simulink model "SMD"  (R2015b)
settings: Solver=VariableStepAuto  StartTime=0.0  StopTime=10.0  RelTol=1e-3
undefined symbols (not defined in the file): a, alpha, alpha_not, alpha_one, b, beta, c, Csfl, Csfr, Csfrl, Csrl, Csrr, d, gama, Ixx, Iyy, Ksfl, Ksfr, Ksrl, Ksrr, Kufl, Kufr, Kurl, Kurr, lamda_not, lamda_one, M, m, Ps, S, tao, Ufl, Ufr, Url, Urr
settings Model: Creator=Guest  LastModifiedBy=Guest

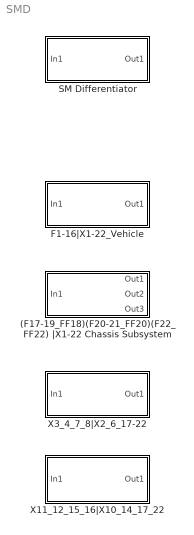
== system SMD ==
  "(F17-19_FF18)(F20-21_FF20)(F22_FF22) |X1-22 Chassis Subsystem " : Subsystem  TreatAsAtomicUnit=on
  "F1-16|X1-22_Vehicle " : Subsystem  TreatAsAtomicUnit=on
  "SM Differentiator " : Subsystem  TreatAsAtomicUnit=on
  X11_12_15_16|X10_14_17_22 : Subsystem  TreatAsAtomicUnit=on
  X3_4_7_8|X2_6_17-22 : Subsystem  TreatAsAtomicUnit=on

== system SMD/(F17-19_FF18)(F20-21_FF20)(F22_FF22) |X1-22 Chassis Subsystem  ==
  In1 : Inport
  F17_18_19_FF18|X1_22 : Subsystem  TreatAsAtomicUnit=on
  "F20_21_FF20|X1_22 " : Subsystem  TreatAsAtomicUnit=on
  F22_FF22|X1_22 : Subsystem  TreatAsAtomicUnit=on
  Out1 : Outport
  Out2 : Outport  Port=2
  Out3 : Outport  Port=3
  wires:
  In1/1 -> F17_18_19_FF18|X1_22/1(In1), "F20_21_FF20|X1_22 "/1(In1), F22_FF22|X1_22/1(In1)
  F22_FF22|X1_22/1(Out1) -> Out3/1
  "F20_21_FF20|X1_22 "/1(Out1) -> Out2/1
  F17_18_19_FF18|X1_22/1(Out1) -> Out1/1

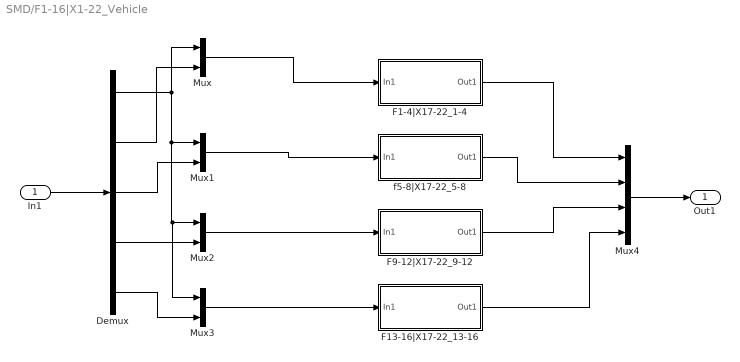
== system SMD/F1-16|X1-22_Vehicle  ==
  In1 : Inport
  Demux : Demux  Outputs=5
  F1-4|X17-22_1-4 : Subsystem  TreatAsAtomicUnit=on
  F13-16|X17-22_13-16 : Subsystem  TreatAsAtomicUnit=on
  F9-12|X17-22_9-12 : Subsystem  TreatAsAtomicUnit=on
  Mux{,1..3} (4 alike) : Mux  Inputs=2
  Mux4 : Mux
  f5-8|X17-22_5-8 : Subsystem  TreatAsAtomicUnit=on
  Out1 : Outport
  wires:
  Demux/1 -> Mux3/1, Mux2/1, Mux1/1, Mux/1
  Demux/2 -> Mux/2
  Mux/1 -> F1-4|X17-22_1-4/1(In1)
  Demux/3 -> Mux1/2
  Mux1/1 -> f5-8|X17-22_5-8/1(In1)
  Demux/4 -> Mux2/2
  Mux2/1 -> F9-12|X17-22_9-12/1(In1)
  Mux3/1 -> F13-16|X17-22_13-16/1(In1)
  Demux/5 -> Mux3/2
  In1/1 -> Demux/1
  F1-4|X17-22_1-4/1(Out1) -> Mux4/1
  f5-8|X17-22_5-8/1(Out1) -> Mux4/2
  F9-12|X17-22_9-12/1(Out1) -> Mux4/3
  F13-16|X17-22_13-16/1(Out1) -> Mux4/4
  Mux4/1 -> Out1/1

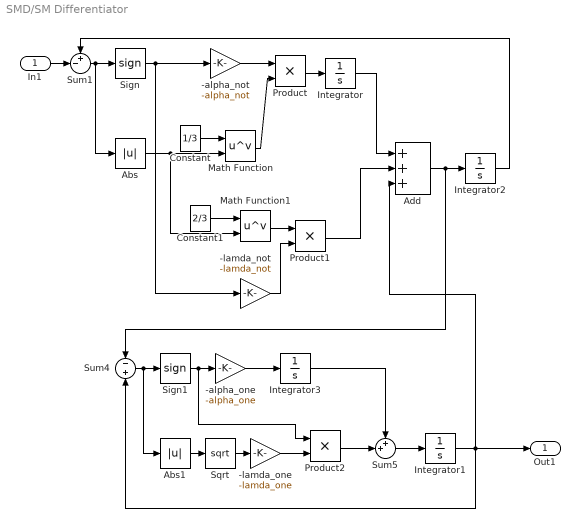
== system SMD/SM Differentiator  ==
  In1 : Inport
  "-alpha_not " : Gain  Gain=-alpha_not
  "-alpha_one " : Gain  Gain=-alpha_one
  "-lamda_not " : Gain  Gain=-lamda_not
  "-lamda_one " : Gain  Gain=-lamda_one
  Abs : Abs
  Abs1 : Abs
  Add : Sum  Inputs=+++
  Constant : Constant  Value=1/3
  Constant1 : Constant  Value=2/3
  Integrator{,1..3} (4 alike) : Integrator
  Math Function : Math  Operator=pow  SaturateOnIntegerOverflow=on
  Math Function1 : Math  Operator=pow  SaturateOnIntegerOverflow=on
  Product : Product
  Product1 : Product
  Product2 : Product
  Sign : Signum
  Sign1 : Signum
  Sqrt : Sqrt  SaturateOnIntegerOverflow=on
  Sum1 : Sum  Inputs=+-|
  Sum4 : Sum  Inputs=-|+
  Sum5 : Sum  Inputs=++|
  Out1 : Outport
  wires:
  Sum1/1 -> Abs/1, Sign/1
  Abs/1 -> Math Function1/2, Math Function/2
  "-alpha_not "/1 -> Product/1
  Constant/1 -> Math Function/1
  Math Function/1 -> Product/2
  Sign/1 -> "-lamda_not "/1, "-alpha_not "/1
  Product/1 -> Integrator/1
  Constant1/1 -> Math Function1/1
  Math Function1/1 -> Product1/1
  "-lamda_not "/1 -> Product1/2
  Integrator/1 -> Add/1
  Product1/1 -> Add/2
  Add/1 -> Sum4/1, Integrator2/1
  Integrator2/1 -> Sum1/1
  Sum4/1 -> Abs1/1, Sign1/1
  Sign1/1 -> Product2/1, "-alpha_one "/1
  "-alpha_one "/1 -> Integrator3/1
  Abs1/1 -> Sqrt/1
  Sqrt/1 -> "-lamda_one "/1
  "-lamda_one "/1 -> Product2/2
  Product2/1 -> Sum5/2
  Integrator3/1 -> Sum5/1
  Sum5/1 -> Integrator1/1
  Integrator1/1 -> Out1/1, Sum4/2, Add/3
  In1/1 -> Sum1/2

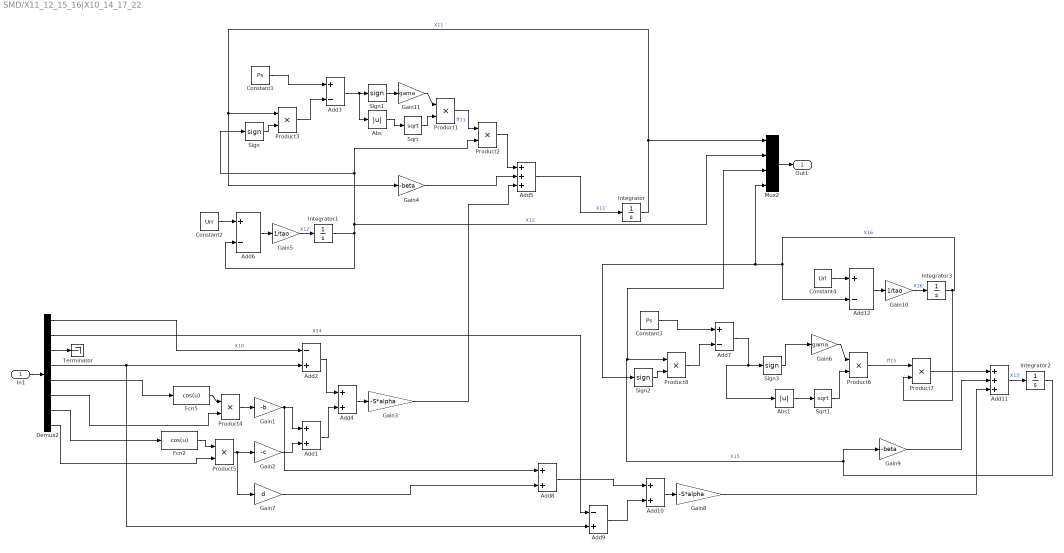
== system SMD/X11_12_15_16|X10_14_17_22 ==
  In1 : Inport
  Abs : Abs
  Abs1 : Abs
  Add{1,4,8,10} (4 alike) : Sum
  Add11 : Sum  Inputs=+++
  Add{3,6..7,12} (4 alike) : Sum  Inputs=+-
  Add2 : Sum  Inputs=-+
  Add5 : Sum  Inputs=+++
  Add9 : Sum  Inputs=-+
  Constant1 : Constant  Value=Ps
  Constant2 : Constant  Value=Urr
  Constant3 : Constant  Value=Ps
  Constant4 : Constant  Value=Url
  Demux2 : Demux  Outputs=8
  Fcn2 : Fcn  Expr=cos(u)
  Fcn5 : Fcn  Expr=cos(u)
  Gain1 : Gain  Gain=-b
  Gain10 : Gain  Gain=1/tao
  Gain11 : Gain  Gain=gama
  Gain2 : Gain  Gain=-c
  Gain3 : Gain  Gain=-S*alpha
  Gain4 : Gain  Gain=-beta
  Gain5 : Gain  Gain=1/tao
  Gain6 : Gain  Gain=gama
  Gain7 : Gain  Gain=d
  Gain8 : Gain  Gain=-S*alpha
  Gain9 : Gain  Gain=-beta
  Integrator{,1..3} (4 alike) : Integrator
  Mux2 : Mux
  Product{1..8} (8 alike) : Product
  Sign{,1..3} (4 alike) : Signum
  Sqrt : Sqrt  SaturateOnIntegerOverflow=on
  Sqrt1 : Sqrt  SaturateOnIntegerOverflow=on
  Terminator : Terminator
  Out1 : Outport
  wires:
  Constant1/1 -> Add3/1
  Product3/1 -> Add3/2
  Add3/1 -> Abs/1, Sign1/1
  Sign1/1 -> Gain11/1
  Abs/1 -> Sqrt/1
  Gain11/1 -> Product1/1
  Sqrt/1 -> Product1/2
  Sign/1 -> Product3/2
  Product1/1 -> Product2/1  "ff11"
  Demux2/5 -> Fcn5/1
  Fcn5/1 -> Product4/1
  Demux2/6 -> Product4/2
  Product4/1 -> Gain1/1
  Demux2/7 -> Fcn2/1
  Fcn2/1 -> Product5/1
  Demux2/8 -> Product5/2
  Product5/1 -> Gain7/1, Gain2/1
  Gain2/1 -> Add1/2
  Gain1/1 -> Add8/1, Add1/1
  Demux2/4 -> Add9/2, Add2/2
  Add2/1 -> Add4/1
  Add1/1 -> Add4/2
  Add4/1 -> Gain3/1
  Product2/1 -> Add5/1
  Gain4/1 -> Add5/2
  Gain3/1 -> Add5/3
  Add5/1 -> Integrator/1  "X11'"
  Integrator/1 -> Gain4/1, Product3/1, Mux2/1  "X11"
  Constant2/1 -> Add6/1
  Add6/1 -> Gain5/1
  Gain5/1 -> Integrator1/1  "X12'"
  Integrator1/1 -> Mux2/2, Sign/1, Product2/2, Add6/2  "X12"
  Constant3/1 -> Add7/1
  Product8/1 -> Add7/2
  Add7/1 -> Abs1/1, Sign3/1
  Sign3/1 -> Gain6/1
  Gain6/1 -> Product6/1
  Sqrt1/1 -> Product6/2
  Sign2/1 -> Product8/2
  Product6/1 -> Product7/1  "ff15"
  Abs1/1 -> Sqrt1/1
  Gain7/1 -> Add8/2
  Demux2/2 -> Add9/1  "X14"
  Add9/1 -> Add10/2
  Add8/1 -> Add10/1
  Add10/1 -> Gain8/1
  Product7/1 -> Add11/1
  Gain9/1 -> Add11/2
  Gain8/1 -> Add11/3
  Add11/1 -> Integrator2/1  "X15'"
  Integrator2/1 -> Mux2/3, Product8/1, Gain9/1  "X15"
  Constant4/1 -> Add12/1
  Add12/1 -> Gain10/1
  Gain10/1 -> Integrator3/1  "X16'"
  Integrator3/1 -> Product7/2, Mux2/4, Sign2/1, Add12/2  "X16"
  Demux2/1 -> Add2/1  "X10"
  Mux2/1 -> Out1/1
  In1/1 -> Demux2/1
  Demux2/3 -> Terminator/1

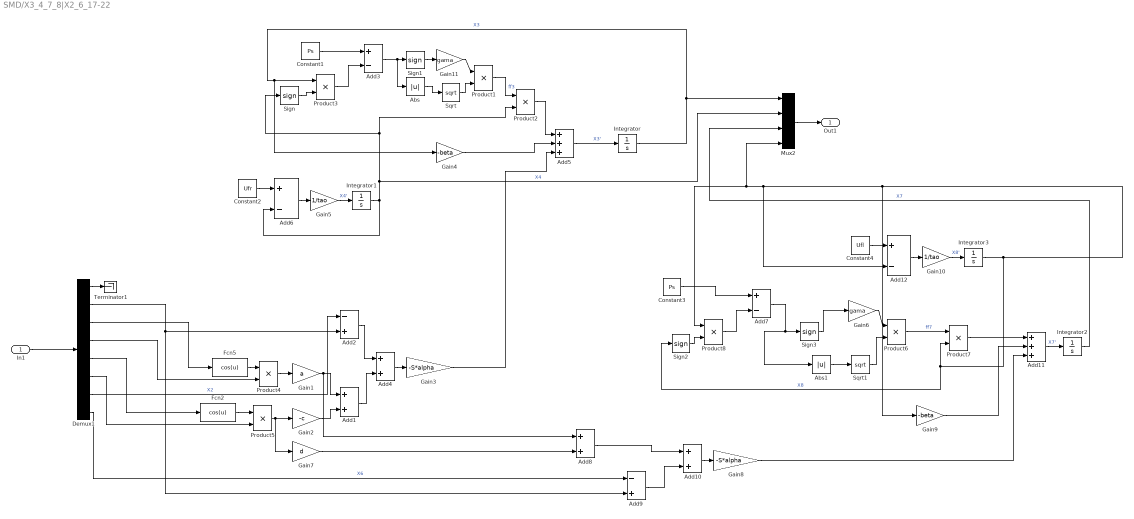
== system SMD/X3_4_7_8|X2_6_17-22 ==
  In1 : Inport
  Abs : Abs
  Abs1 : Abs
  Add{1,4,8,10} (4 alike) : Sum
  Add11 : Sum  Inputs=+++
  Add{3,6..7,12} (4 alike) : Sum  Inputs=+-
  Add2 : Sum  Inputs=-+
  Add5 : Sum  Inputs=+++
  Add9 : Sum  Inputs=-+
  Constant1 : Constant  Value=Ps
  Constant2 : Constant  Value=Ufr
  Constant3 : Constant  Value=Ps
  Constant4 : Constant  Value=Ufl
  Demux1 : Demux  Outputs=8
  Fcn2 : Fcn  Expr=cos(u)
  Fcn5 : Fcn  Expr=cos(u)
  Gain1 : Gain  Gain=a
  Gain10 : Gain  Gain=1/tao
  Gain11 : Gain  Gain=gama
  Gain2 : Gain  Gain=-c
  Gain3 : Gain  Gain=-S*alpha
  Gain4 : Gain  Gain=-beta
  Gain5 : Gain  Gain=1/tao
  Gain6 : Gain  Gain=gama
  Gain7 : Gain  Gain=d
  Gain8 : Gain  Gain=-S*alpha
  Gain9 : Gain  Gain=-beta
  Integrator{,1..3} (4 alike) : Integrator
  Mux2 : Mux
  Product{1..8} (8 alike) : Product
  Sign{,1..3} (4 alike) : Signum
  Sqrt : Sqrt  SaturateOnIntegerOverflow=on
  Sqrt1 : Sqrt  SaturateOnIntegerOverflow=on
  Terminator1 : Terminator
  Out1 : Outport
  wires:
  Constant1/1 -> Add3/1
  Product3/1 -> Add3/2
  Add3/1 -> Abs/1, Sign1/1
  Sign1/1 -> Gain11/1
  Abs/1 -> Sqrt/1
  Gain11/1 -> Product1/1
  Sqrt/1 -> Product1/2
  Sign/1 -> Product3/2
  Product1/1 -> Product2/1  "ff3"
  Demux1/3 -> Fcn5/1
  Fcn5/1 -> Product4/1
  Demux1/4 -> Product4/2
  Product4/1 -> Gain1/1
  Fcn2/1 -> Product5/1
  Product5/1 -> Gain7/1, Gain2/1
  Gain2/1 -> Add1/2
  Gain1/1 -> Add8/1, Add1/1
  Demux1/2 -> Add9/2, Add2/2
  Demux1/7 -> Add2/1  "X2"
  Add2/1 -> Add4/1
  Add1/1 -> Add4/2
  Add4/1 -> Gain3/1
  Product2/1 -> Add5/1
  Gain4/1 -> Add5/2
  Gain3/1 -> Add5/3
  Add5/1 -> Integrator/1  "X3'"
  Constant2/1 -> Add6/1
  Add6/1 -> Gain5/1
  Gain5/1 -> Integrator1/1  "X4'"
  Constant3/1 -> Add7/1
  Product8/1 -> Add7/2
  Add7/1 -> Abs1/1, Sign3/1
  Sign3/1 -> Gain6/1
  Gain6/1 -> Product6/1
  Sqrt1/1 -> Product6/2
  Sign2/1 -> Product8/2
  Product6/1 -> Product7/1  "ff7"
  Abs1/1 -> Sqrt1/1
  Gain7/1 -> Add8/2
  Add9/1 -> Add10/2
  Add8/1 -> Add10/1
  Add10/1 -> Gain8/1
  Product7/1 -> Add11/1
  Gain9/1 -> Add11/2
  Gain8/1 -> Add11/3
  Add11/1 -> Integrator2/1  "X7'"
  Integrator3/1 -> Product7/2, Sign2/1, Gain9/1, Add12/2, Product8/1, Mux2/4  "X8"
  Constant4/1 -> Add12/1
  Add12/1 -> Gain10/1
  Gain10/1 -> Integrator3/1  "X8'"
  Integrator2/1 -> Mux2/3  "X7"
  Integrator/1 -> Mux2/1, Gain4/1, Product3/1  "X3"
  Integrator1/1 -> Mux2/2, Sign/1, Product2/2, Add6/2  "X4"
  Demux1/8 -> Add9/1  "X6"
  In1/1 -> Demux1/1
  Mux2/1 -> Out1/1
  Demux1/1 -> Terminator1/1
  Demux1/5 -> Fcn2/1
  Demux1/6 -> Product5/2

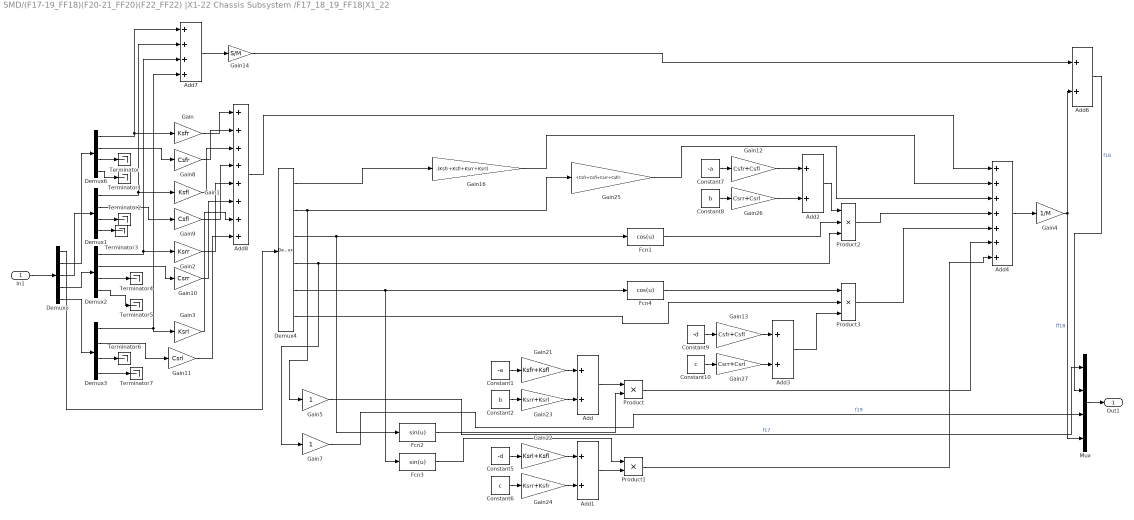
== system SMD/(F17-19_FF18)(F20-21_FF20)(F22_FF22) |X1-22 Chassis Subsystem /F17_18_19_FF18|X1_22 ==
  In1 : Inport
  Add{,1..3,6} (5 alike) : Sum
  Add4 : Sum  Inputs=+++++++
  Add7 : Sum  Inputs=++++
  Add8 : Sum  Inputs=++++++++
  Constant1 : Constant  Value=-a
  Constant10 : Constant  Value=c
  Constant2 : Constant  Value=b
  Constant5 : Constant  Value=-d
  Constant6 : Constant  Value=c
  Constant7 : Constant  Value=-a
  Constant8 : Constant  Value=b
  Constant9 : Constant  Value=-d
  Demux{1..3,6} (4 alike) : Demux
  Demux4 : Demux  Outputs=6
  Demux5 : Demux  Outputs=5
  Fcn1 : Fcn  Expr=cos(u)
  Fcn2 : Fcn  Expr=sin(u)
  Fcn3 : Fcn  Expr=sin(u)
  Fcn4 : Fcn  Expr=cos(u)
  Gain : Gain  Gain=Ksfr
  Gain1 : Gain  Gain=Ksfl
  Gain10 : Gain  Gain=Csrr
  Gain11 : Gain  Gain=Csrl
  Gain12 : Gain  Gain=Csfr+Csfl
  Gain13 : Gain  Gain=Csfr+Csfl
  Gain14 : Gain  Gain=S/M
  Gain16 : Gain  Gain=-(Ksfr+Ksfl+Ksrr+Ksrl)
  Gain2 : Gain  Gain=Ksrr
  Gain21 : Gain  Gain=Ksfr+Ksfl
  Gain22 : Gain  Gain=Ksrl+Ksfl
  Gain23 : Gain  Gain=Ksrr+Ksrl
  Gain24 : Gain  Gain=Ksrr+Ksfr
  Gain25 : Gain  Gain=-(Csfr+Csfl+Csrr+Csfr)
  Gain26 : Gain  Gain=Csrr+Csrl
  Gain27 : Gain  Gain=Csrr+Csrl
  Gain3 : Gain  Gain=Ksrl
  Gain4 : Gain  Gain=1/M
  Gain5 : Gain
  Gain7 : Gain
  Gain8 : Gain  Gain=Csfr
  Gain9 : Gain  Gain=Csfl
  Mux : Mux
  Product : Product
  Product1 : Product
  Product2 : Product  Inputs=3
  Product3 : Product  Inputs=3
  Terminator{,1..7} (8 alike) : Terminator
  Out1 : Outport
  wires:
  Demux6/1 -> Add7/1, Gain/1
  Demux1/1 -> Gain1/1, Add7/2
  Demux2/1 -> Gain2/1, Add7/3
  Demux3/1 -> Gain3/1, Add7/4
  Demux4/1 -> Gain16/1
  Demux4/3 -> Fcn2/1, Fcn1/1
  Gain21/1 -> Add/1
  Constant1/1 -> Gain21/1
  Gain23/1 -> Add/2
  Constant2/1 -> Gain23/1
  Add/1 -> Product/1
  Fcn2/1 -> Product/2
  Demux4/5 -> Fcn3/1, Fcn4/1
  Gain22/1 -> Add1/1
  Gain24/1 -> Add1/2
  Constant5/1 -> Gain22/1
  Constant6/1 -> Gain24/1
  Add1/1 -> Product1/2
  Fcn3/1 -> Product1/1
  Demux4/2 -> Gain5/1, Gain25/1
  Demux4/4 -> Gain7/1, Product2/3
  Fcn1/1 -> Product2/2
  Gain12/1 -> Add2/1
  Constant7/1 -> Gain12/1
  Gain26/1 -> Add2/2
  Constant8/1 -> Gain26/1
  Add2/1 -> Product2/1
  Gain13/1 -> Add3/1
  Constant9/1 -> Gain13/1
  Gain27/1 -> Add3/2
  Constant10/1 -> Gain27/1
  Fcn4/1 -> Product3/1
  Demux4/6 -> Product3/2
  Add3/1 -> Product3/3
  Product/1 -> Add4/6
  Product1/1 -> Add4/7
  Add4/1 -> Gain4/1
  Gain14/1 -> Add6/1
  Gain4/1 -> Add6/2, Mux/4  "ff18"
  Add6/1 -> Mux/2  "f18"
  Gain5/1 -> Mux/1  "f17"
  Gain7/1 -> Mux/3  "f19"
  Demux6/2 -> Gain8/1
  Demux1/2 -> Gain9/1
  Demux2/2 -> Gain10/1
  Demux3/2 -> Gain11/1
  Add7/1 -> Gain14/1
  Gain/1 -> Add8/1
  Gain8/1 -> Add8/2
  Gain1/1 -> Add8/3
  Gain9/1 -> Add8/4
  Gain2/1 -> Add8/5
  Gain10/1 -> Add8/6
  Gain3/1 -> Add8/7
  Gain11/1 -> Add8/8
  Product3/1 -> Add4/5
  Product2/1 -> Add4/4
  Gain25/1 -> Add4/3
  Gain16/1 -> Add4/2
  Add8/1 -> Add4/1
  Demux6/3 -> Terminator/1
  Demux6/4 -> Terminator1/1
  Demux1/3 -> Terminator2/1
  Demux1/4 -> Terminator3/1
  Demux2/3 -> Terminator4/1
  Demux2/4 -> Terminator5/1
  Demux3/3 -> Terminator6/1
  Demux3/4 -> Terminator7/1
  Demux5/2 -> Demux6/1
  Demux5/3 -> Demux1/1
  Demux5/4 -> Demux2/1
  Demux5/5 -> Demux3/1
  In1/1 -> Demux5/1
  Mux/1 -> Out1/1
  Demux5/1 -> Demux4/1

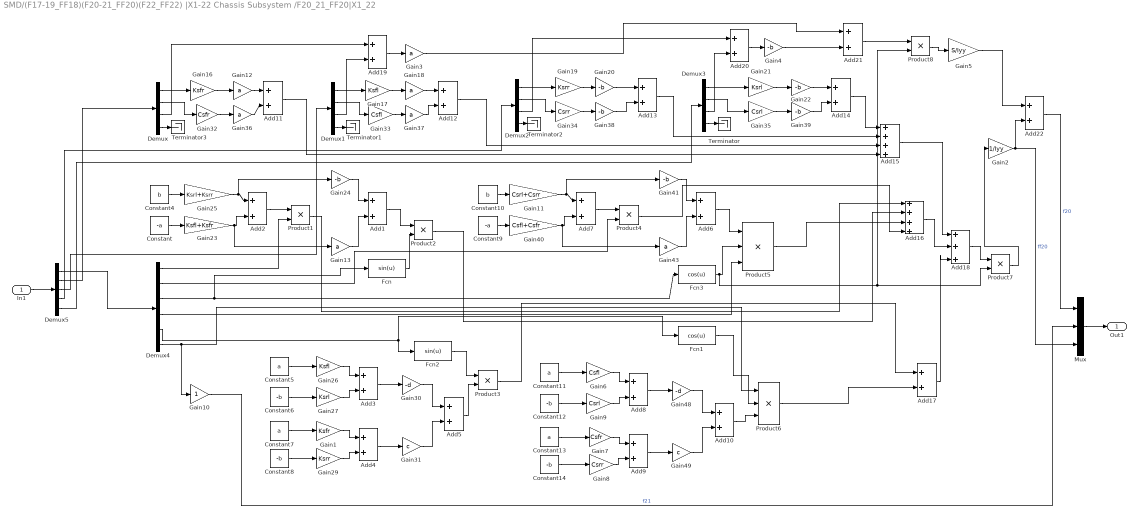
== system SMD/(F17-19_FF18)(F20-21_FF20)(F22_FF22) |X1-22 Chassis Subsystem /F20_21_FF20|X1_22  ==
  In1 : Inport
  Add{1..14,17,19..22} (19 alike) : Sum
  Add15 : Sum  Inputs=++++
  Add16 : Sum  Inputs=++++
  Add18 : Sum  Inputs=+++
  Constant : Constant  Value=-a
  Constant10 : Constant  Value=b
  Constant{5,7,11,13} (4 alike) : Constant  Value=a
  Constant{6,8,12,14} (4 alike) : Constant  Value=-b
  Constant4 : Constant  Value=b
  Constant9 : Constant  Value=-a
  Demux{,1..3} (4 alike) : Demux
  Demux4 : Demux  Outputs=6
  Demux5 : Demux  Outputs=5
  Fcn : Fcn  Expr=sin(u)
  Fcn1 : Fcn  Expr=cos(u)
  Fcn2 : Fcn  Expr=sin(u)
  Fcn3 : Fcn  Expr=cos(u)
  Gain1 : Gain  Gain=Ksfr
  Gain10 : Gain
  Gain11 : Gain  Gain=Csrl+Csrr
  Gain{3,12..13,18,36..37,43} (7 alike) : Gain  Gain=a
  Gain16 : Gain  Gain=Ksfr
  Gain17 : Gain  Gain=Ksfl
  Gain19 : Gain  Gain=Ksrr
  Gain2 : Gain  Gain=1/Iyy
  Gain{4,20,22,24,38..39,41} (7 alike) : Gain  Gain=-b
  Gain21 : Gain  Gain=Ksrl
  Gain23 : Gain  Gain=Ksfl+Ksfr
  Gain25 : Gain  Gain=Ksrl+Ksrr
  Gain26 : Gain  Gain=Ksfl
  Gain27 : Gain  Gain=Ksrl
  Gain29 : Gain  Gain=Ksrr
  Gain30 : Gain  Gain=-d
  Gain31 : Gain  Gain=c
  Gain32 : Gain  Gain=Csfr
  Gain33 : Gain  Gain=Csfl
  Gain34 : Gain  Gain=Csrr
  Gain35 : Gain  Gain=Csrl
  Gain40 : Gain  Gain=Csfl+Csfr
  Gain48 : Gain  Gain=-d
  Gain49 : Gain  Gain=c
  Gain5 : Gain  Gain=S/Iyy
  Gain6 : Gain  Gain=Csfl
  Gain7 : Gain  Gain=Csfr
  Gain8 : Gain  Gain=Csrr
  Gain9 : Gain  Gain=Csrl
  Mux : Mux  Inputs=3
  Product{1..4,7..8} (6 alike) : Product
  Product5 : Product  Inputs=3
  Product6 : Product  Inputs=3
  Terminator{,1..3} (4 alike) : Terminator
  Out1 : Outport
  wires:
  Demux/1 -> Gain16/1
  Gain16/1 -> Gain12/1
  Demux1/1 -> Gain17/1
  Gain17/1 -> Gain18/1
  Demux2/1 -> Gain19/1
  Gain19/1 -> Gain20/1
  Demux3/1 -> Gain21/1
  Gain21/1 -> Gain22/1
  Constant/1 -> Gain23/1
  Constant4/1 -> Gain25/1
  Gain23/1 -> Gain13/1, Add2/2
  Gain25/1 -> Gain24/1, Add2/1
  Add2/1 -> Product1/1
  Demux4/1 -> Product1/2
  Gain24/1 -> Add1/1
  Gain13/1 -> Add1/2
  Constant5/1 -> Gain26/1
  Constant6/1 -> Gain27/1
  Gain26/1 -> Add3/1
  Gain27/1 -> Add3/2
  Constant8/1 -> Gain29/1
  Constant7/1 -> Gain1/1
  Gain1/1 -> Add4/1
  Gain29/1 -> Add4/2
  Add3/1 -> Gain30/1
  Add4/1 -> Gain31/1
  Demux4/3 -> Fcn3/1, Fcn/1
  Add1/1 -> Product2/1
  Fcn/1 -> Product2/2
  Demux4/5 -> Fcn1/1, Fcn2/1
  Gain30/1 -> Add5/1
  Gain31/1 -> Add5/2
  Add5/1 -> Product3/2
  Fcn2/1 -> Product3/1
  Demux/2 -> Gain32/1
  Demux1/2 -> Gain33/1
  Demux2/2 -> Gain34/1
  Demux3/2 -> Gain35/1
  Gain32/1 -> Gain36/1
  Gain33/1 -> Gain37/1
  Gain34/1 -> Gain38/1
  Gain35/1 -> Gain39/1
  Constant10/1 -> Gain11/1
  Gain40/1 -> Gain43/1, Add7/2
  Gain11/1 -> Add7/1, Gain41/1
  Add7/1 -> Product4/1
  Demux4/2 -> Product4/2
  Gain41/1 -> Add6/1
  Gain43/1 -> Add6/2
  Add6/1 -> Product5/1
  Constant9/1 -> Gain40/1
  Fcn3/1 -> Product8/2, Product7/2, Product5/2
  Demux4/4 -> Product5/3
  Constant11/1 -> Gain6/1
  Constant12/1 -> Gain9/1
  Gain6/1 -> Add8/1
  Gain9/1 -> Add8/2
  Constant14/1 -> Gain8/1
  Constant13/1 -> Gain7/1
  Gain7/1 -> Add9/1
  Add8/1 -> Gain48/1
  Add9/1 -> Gain49/1
  Gain48/1 -> Add10/1
  Gain49/1 -> Add10/2
  Add10/1 -> Product6/3
  Fcn1/1 -> Product6/2
  Gain8/1 -> Add9/2
  Demux4/6 -> Gain10/1, Product6/1
  Gain12/1 -> Add11/1
  Gain36/1 -> Add11/2
  Gain18/1 -> Add12/1
  Gain37/1 -> Add12/2
  Gain20/1 -> Add13/1
  Gain38/1 -> Add13/2
  Gain22/1 -> Add14/1
  Gain39/1 -> Add14/2
  Add14/1 -> Add15/1
  Add13/1 -> Add15/2
  Add12/1 -> Add15/3
  Add11/1 -> Add15/4
  Product1/1 -> Add16/1
  Product2/1 -> Add16/2
  Product5/1 -> Add16/3
  Product4/1 -> Add16/4
  Product3/1 -> Add17/1
  Product6/1 -> Add17/2
  Add15/1 -> Add18/1
  Add17/1 -> Add18/3
  Add16/1 -> Add18/2
  Add18/1 -> Product7/1
  Product7/1 -> Gain2/1
  Demux/3 -> Add19/1
  Demux1/3 -> Add19/2
  Add19/1 -> Gain3/1
  Demux2/3 -> Add20/1
  Demux3/3 -> Add20/2
  Add20/1 -> Gain4/1
  Gain4/1 -> Add21/2
  Gain3/1 -> Add21/1
  Add21/1 -> Product8/1
  Product8/1 -> Gain5/1
  Gain5/1 -> Add22/1
  Gain2/1 -> Mux/3, Add22/2  "ff20"
  Gain10/1 -> Mux/2  "f21"
  Add22/1 -> Mux/1  "f20"
  Demux1/4 -> Terminator1/1
  Demux2/4 -> Terminator2/1
  Demux3/4 -> Terminator/1
  Demux/4 -> Terminator3/1
  Demux5/1 -> Demux4/1
  Demux5/2 -> Demux/1
  Demux5/3 -> Demux1/1
  Demux5/4 -> Demux2/1
  Demux5/5 -> Demux3/1
  In1/1 -> Demux5/1
  Mux/1 -> Out1/1

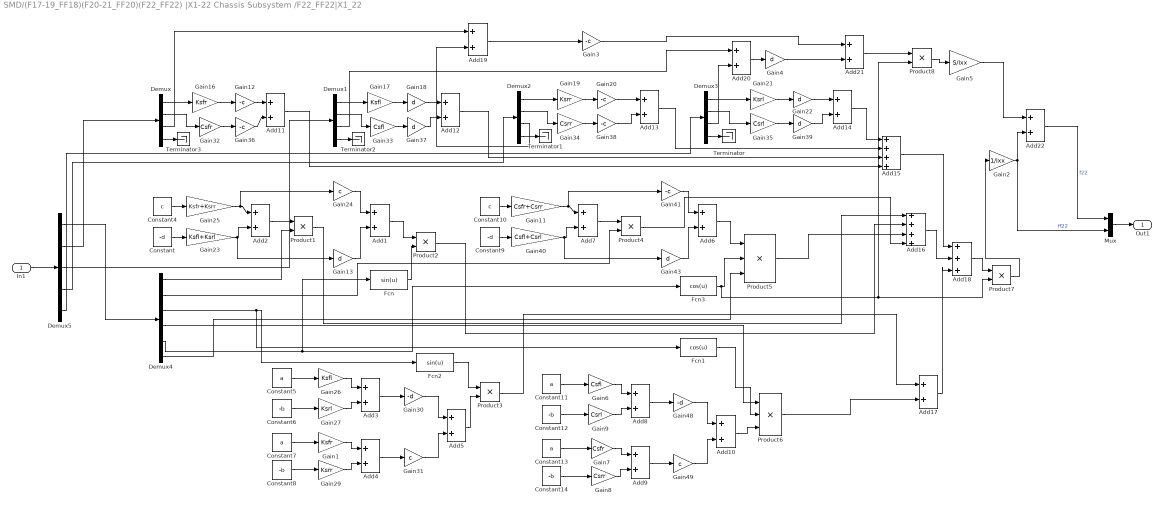
== system SMD/(F17-19_FF18)(F20-21_FF20)(F22_FF22) |X1-22 Chassis Subsystem /F22_FF22|X1_22 ==
  In1 : Inport
  Add{1..14,17,19..22} (19 alike) : Sum
  Add15 : Sum  Inputs=++++
  Add16 : Sum  Inputs=++++
  Add18 : Sum  Inputs=+++
  Constant : Constant  Value=-d
  Constant10 : Constant  Value=c
  Constant{5,7,11,13} (4 alike) : Constant  Value=a
  Constant{6,8,12,14} (4 alike) : Constant  Value=-b
  Constant4 : Constant  Value=c
  Constant9 : Constant  Value=-d
  Demux{,1..3} (4 alike) : Demux
  Demux4 : Demux  Outputs=6
  Demux5 : Demux  Outputs=5
  Fcn : Fcn  Expr=sin(u)
  Fcn1 : Fcn  Expr=cos(u)
  Fcn2 : Fcn  Expr=sin(u)
  Fcn3 : Fcn  Expr=cos(u)
  Gain1 : Gain  Gain=Ksfr
  Gain11 : Gain  Gain=Csfr+Csrr
  Gain{3,12,20,36,38,41} (6 alike) : Gain  Gain=-c
  Gain{4,13,18,22,37,39,43} (7 alike) : Gain  Gain=d
  Gain16 : Gain  Gain=Ksfr
  Gain17 : Gain  Gain=Ksfl
  Gain19 : Gain  Gain=Ksrr
  Gain2 : Gain  Gain=1/Ixx
  Gain21 : Gain  Gain=Ksrl
  Gain23 : Gain  Gain=Ksfl+Ksrl
  Gain24 : Gain  Gain=c
  Gain25 : Gain  Gain=Ksfr+Ksrr
  Gain26 : Gain  Gain=Ksfl
  Gain27 : Gain  Gain=Ksrl
  Gain29 : Gain  Gain=Ksrr
  Gain30 : Gain  Gain=-d
  Gain31 : Gain  Gain=c
  Gain32 : Gain  Gain=Csfr
  Gain33 : Gain  Gain=Csfl
  Gain34 : Gain  Gain=Csrr
  Gain35 : Gain  Gain=Csrl
  Gain40 : Gain  Gain=Csfl+Csrl
  Gain48 : Gain  Gain=-d
  Gain49 : Gain  Gain=c
  Gain5 : Gain  Gain=S/Ixx
  Gain6 : Gain  Gain=Csfl
  Gain7 : Gain  Gain=Csfr
  Gain8 : Gain  Gain=Csrr
  Gain9 : Gain  Gain=Csrl
  Mux : Mux  Inputs=2
  Product{1..4,7..8} (6 alike) : Product
  Product5 : Product  Inputs=3
  Product6 : Product  Inputs=3
  Terminator{,1..3} (4 alike) : Terminator
  Out1 : Outport
  wires:
  Demux/1 -> Gain16/1
  Gain16/1 -> Gain12/1
  Demux1/1 -> Gain17/1
  Gain17/1 -> Gain18/1
  Demux2/1 -> Gain19/1
  Gain19/1 -> Gain20/1
  Demux3/1 -> Gain21/1
  Gain21/1 -> Gain22/1
  Constant/1 -> Gain23/1
  Constant4/1 -> Gain25/1
  Gain23/1 -> Gain13/1, Add2/2
  Gain25/1 -> Gain24/1, Add2/1
  Add2/1 -> Product1/1
  Demux4/1 -> Product1/2
  Gain24/1 -> Add1/1
  Gain13/1 -> Add1/2
  Constant5/1 -> Gain26/1
  Constant6/1 -> Gain27/1
  Gain26/1 -> Add3/1
  Gain27/1 -> Add3/2
  Constant8/1 -> Gain29/1
  Constant7/1 -> Gain1/1
  Gain1/1 -> Add4/1
  Gain29/1 -> Add4/2
  Add3/1 -> Gain30/1
  Add4/1 -> Gain31/1
  Demux4/3 -> Fcn1/1, Fcn2/1
  Add1/1 -> Product2/1
  Fcn/1 -> Product2/2
  Demux4/5 -> Fcn/1, Fcn3/1
  Gain30/1 -> Add5/1
  Gain31/1 -> Add5/2
  Add5/1 -> Product3/2
  Fcn2/1 -> Product3/1
  Demux/2 -> Gain32/1
  Demux1/2 -> Gain33/1
  Demux2/2 -> Gain34/1
  Demux3/2 -> Gain35/1
  Gain32/1 -> Gain36/1
  Gain33/1 -> Gain37/1
  Gain34/1 -> Gain38/1
  Gain35/1 -> Gain39/1
  Constant10/1 -> Gain11/1
  Gain40/1 -> Gain43/1, Add7/2
  Gain11/1 -> Add7/1, Gain41/1
  Add7/1 -> Product4/1
  Demux4/2 -> Product4/2
  Gain41/1 -> Add6/1
  Gain43/1 -> Add6/2
  Add6/1 -> Product5/1
  Constant9/1 -> Gain40/1
  Fcn3/1 -> Product8/2, Product7/2, Product5/2
  Constant11/1 -> Gain6/1
  Constant12/1 -> Gain9/1
  Gain6/1 -> Add8/1
  Gain9/1 -> Add8/2
  Constant14/1 -> Gain8/1
  Constant13/1 -> Gain7/1
  Gain7/1 -> Add9/1
  Add8/1 -> Gain48/1
  Add9/1 -> Gain49/1
  Gain48/1 -> Add10/1
  Gain49/1 -> Add10/2
  Add10/1 -> Product6/3
  Fcn1/1 -> Product6/2
  Gain8/1 -> Add9/2
  Demux4/6 -> Product5/3
  Gain12/1 -> Add11/1
  Gain36/1 -> Add11/2
  Gain18/1 -> Add12/1
  Gain37/1 -> Add12/2
  Gain20/1 -> Add13/1
  Gain38/1 -> Add13/2
  Gain22/1 -> Add14/1
  Gain39/1 -> Add14/2
  Add14/1 -> Add15/1
  Add13/1 -> Add15/2
  Add12/1 -> Add15/3
  Add11/1 -> Add15/4
  Product1/1 -> Add16/1
  Product2/1 -> Add16/2
  Product5/1 -> Add16/3
  Product4/1 -> Add16/4
  Product3/1 -> Add17/1
  Product6/1 -> Add17/2
  Add15/1 -> Add18/1
  Add17/1 -> Add18/3
  Add16/1 -> Add18/2
  Add18/1 -> Product7/1
  Product7/1 -> Gain2/1
  Demux/3 -> Add19/1
  Add19/1 -> Gain3/1
  Add20/1 -> Gain4/1
  Gain4/1 -> Add21/2
  Gain3/1 -> Add21/1
  Add21/1 -> Product8/1
  Product8/1 -> Gain5/1
  Gain5/1 -> Add22/1
  Gain2/1 -> Add22/2, Mux/2  "ff22"
  Add22/1 -> Mux/1  "f22"
  Demux4/4 -> Product6/1
  Demux2/3 -> Add19/2
  Demux1/3 -> Add20/1
  Demux3/3 -> Add20/2
  Demux5/1 -> Demux4/1
  Demux5/2 -> Demux/1
  Demux5/3 -> Demux1/1
  Demux5/4 -> Demux2/1
  Demux5/5 -> Demux3/1
  Demux3/4 -> Terminator/1
  Demux2/4 -> Terminator1/1
  Demux1/4 -> Terminator2/1
  Demux/4 -> Terminator3/1
  In1/1 -> Demux5/1
  Mux/1 -> Out1/1

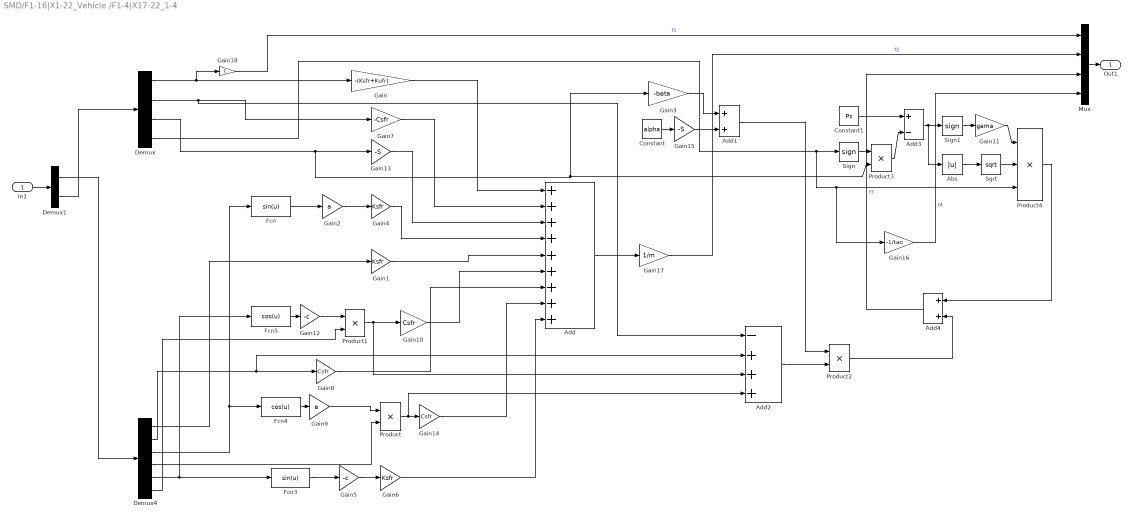
== system SMD/F1-16|X1-22_Vehicle /F1-4|X17-22_1-4 ==
  In1 : Inport
  Abs : Abs
  Add : Sum  Inputs=+++++++++
  Add1 : Sum
  Add2 : Sum  Inputs=-+++
  Add3 : Sum  Inputs=+-
  Add4 : Sum
  Constant : Constant  Value=alpha
  Constant1 : Constant  Value=Ps
  Demux : Demux
  Demux1 : Demux  Outputs=2
  Demux4 : Demux  Outputs=6
  Fcn : Fcn  Expr=sin(u)
  Fcn3 : Fcn  Expr=sin(u)
  Fcn4 : Fcn  Expr=cos(u)
  Fcn5 : Fcn  Expr=cos(u)
  Gain : Gain  Gain=-(Ksfr+Kufr)
  Gain1 : Gain  Gain=Ksfr
  Gain10 : Gain  Gain=Csfr
  Gain11 : Gain  Gain=gama
  Gain12 : Gain  Gain=-c
  Gain13 : Gain  Gain=-S
  Gain14 : Gain  Gain=Csfr
  Gain15 : Gain  Gain=-S
  Gain16 : Gain  Gain=-1/tao
  Gain17 : Gain  Gain=1/m
  Gain18 : Gain
  Gain2 : Gain  Gain=a
  Gain3 : Gain  Gain=-beta
  Gain4 : Gain  Gain=Ksfr
  Gain5 : Gain  Gain=-c
  Gain6 : Gain  Gain=Ksfr
  Gain7 : Gain  Gain=-Csfr
  Gain8 : Gain  Gain=Csfr
  Gain9 : Gain  Gain=a
  Mux : Mux
  Product{,1..3} (4 alike) : Product
  Product4 : Product  Inputs=3
  Sign : Signum
  Sign1 : Signum
  Sqrt : Sqrt  SaturateOnIntegerOverflow=on
  Out1 : Outport
  wires:
  Demux/1 -> Gain18/1, Gain/1
  Demux4/1 -> Gain1/1
  Demux4/3 -> Fcn/1, Fcn4/1
  Fcn/1 -> Gain2/1
  Gain2/1 -> Gain4/1
  Demux4/5 -> Fcn5/1, Fcn3/1
  Fcn3/1 -> Gain5/1
  Gain5/1 -> Gain6/1
  Demux/2 -> Add2/1, Gain7/1
  Demux4/2 -> Add2/2, Gain8/1
  Fcn4/1 -> Gain9/1
  Gain9/1 -> Product/1
  Demux4/4 -> Product/2
  Fcn5/1 -> Gain12/1
  Demux4/6 -> Product1/2
  Gain12/1 -> Product1/1
  Demux/3 -> Gain3/1, Product3/2, Gain13/1
  Gain/1 -> Add/1
  Gain7/1 -> Add/2
  Gain13/1 -> Add/3
  Gain4/1 -> Add/4
  Gain1/1 -> Add/5
  Product1/1 -> Add2/3, Gain10/1
  Gain8/1 -> Add/7
  Product/1 -> Add2/4, Gain14/1
  Gain6/1 -> Add/9
  Constant/1 -> Gain15/1
  Gain3/1 -> Add1/1
  Gain15/1 -> Add1/2
  Gain14/1 -> Add/8
  Gain10/1 -> Add/6
  Add2/1 -> Product2/2
  Add1/1 -> Product2/1
  Demux/4 -> Gain16/1, Product4/3, Sign/1
  Sign/1 -> Product3/1
  Constant1/1 -> Add3/1
  Product3/1 -> Add3/2
  Add3/1 -> Abs/1, Sign1/1
  Sign1/1 -> Gain11/1
  Abs/1 -> Sqrt/1
  Gain11/1 -> Product4/1
  Sqrt/1 -> Product4/2
  Product2/1 -> Add4/2
  Add/1 -> Gain17/1
  Gain17/1 -> Mux/2  "f2"
  Product4/1 -> Add4/1
  Gain18/1 -> Mux/1  "f1"
  Add4/1 -> Mux/3  "f3"
  Gain16/1 -> Mux/4  "f4"
  Mux/1 -> Out1/1
  Demux1/1 -> Demux4/1
  In1/1 -> Demux1/1
  Demux1/2 -> Demux/1

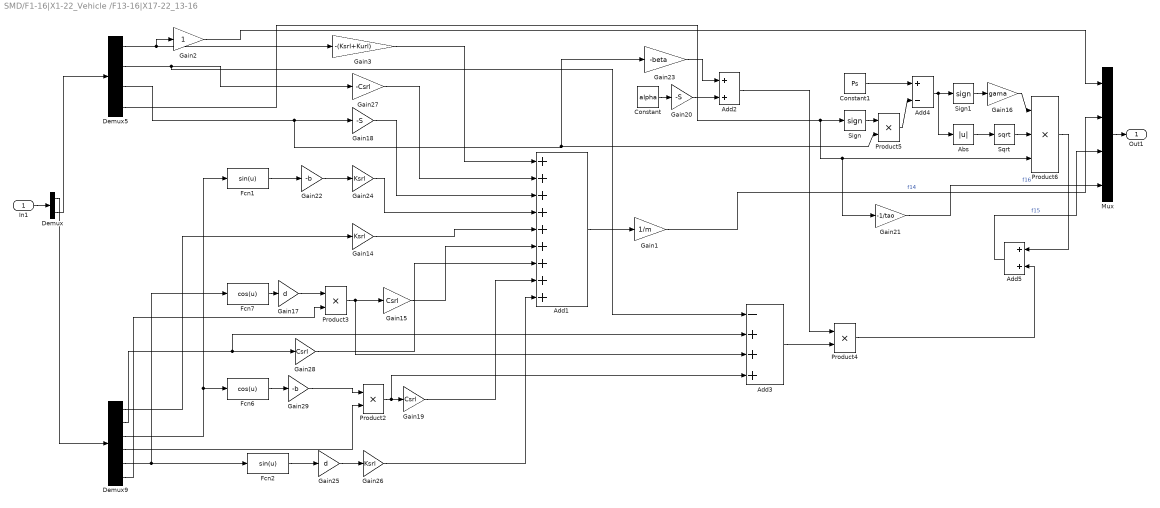
== system SMD/F1-16|X1-22_Vehicle /F13-16|X17-22_13-16 ==
  In1 : Inport
  Abs : Abs
  Add1 : Sum  Inputs=+++++++++
  Add2 : Sum
  Add3 : Sum  Inputs=-+++
  Add4 : Sum  Inputs=+-
  Add5 : Sum
  Constant : Constant  Value=alpha
  Constant1 : Constant  Value=Ps
  Demux : Demux  Outputs=2
  Demux5 : Demux
  Demux9 : Demux  Outputs=6
  Fcn1 : Fcn  Expr=sin(u)
  Fcn2 : Fcn  Expr=sin(u)
  Fcn6 : Fcn  Expr=cos(u)
  Fcn7 : Fcn  Expr=cos(u)
  Gain1 : Gain  Gain=1/m
  Gain14 : Gain  Gain=Ksrl
  Gain15 : Gain  Gain=Csrl
  Gain16 : Gain  Gain=gama
  Gain17 : Gain  Gain=d
  Gain18 : Gain  Gain=-S
  Gain19 : Gain  Gain=Csrl
  Gain2 : Gain
  Gain20 : Gain  Gain=-S
  Gain21 : Gain  Gain=-1/tao
  Gain22 : Gain  Gain=-b
  Gain23 : Gain  Gain=-beta
  Gain24 : Gain  Gain=Ksrl
  Gain25 : Gain  Gain=d
  Gain26 : Gain  Gain=Ksrl
  Gain27 : Gain  Gain=-Csrl
  Gain28 : Gain  Gain=Csrl
  Gain29 : Gain  Gain=-b
  Gain3 : Gain  Gain=-(Ksrl+Kurl)
  Mux : Mux
  Product{2..5} (4 alike) : Product
  Product6 : Product  Inputs=3
  Sign : Signum
  Sign1 : Signum
  Sqrt : Sqrt  SaturateOnIntegerOverflow=on
  Out1 : Outport
  wires:
  Demux5/1 -> Gain2/1, Gain3/1
  Demux9/1 -> Gain14/1
  Demux9/3 -> Fcn1/1, Fcn6/1
  Fcn1/1 -> Gain22/1
  Gain22/1 -> Gain24/1
  Demux9/5 -> Fcn7/1, Fcn2/1
  Fcn2/1 -> Gain25/1
  Gain25/1 -> Gain26/1
  Demux5/2 -> Add3/1, Gain27/1
  Demux9/2 -> Add3/2, Gain28/1
  Fcn6/1 -> Gain29/1
  Gain29/1 -> Product2/1
  Demux9/4 -> Product2/2
  Fcn7/1 -> Gain17/1
  Demux9/6 -> Product3/2
  Gain17/1 -> Product3/1
  Demux5/3 -> Gain23/1, Product5/2, Gain18/1
  Gain3/1 -> Add1/1
  Gain27/1 -> Add1/2
  Gain18/1 -> Add1/3
  Gain24/1 -> Add1/4
  Gain14/1 -> Add1/5
  Product3/1 -> Add3/3, Gain15/1
  Gain28/1 -> Add1/7
  Product2/1 -> Add3/4, Gain19/1
  Gain26/1 -> Add1/9
  Constant/1 -> Gain20/1
  Gain23/1 -> Add2/1
  Gain20/1 -> Add2/2
  Gain19/1 -> Add1/8
  Gain15/1 -> Add1/6
  Add3/1 -> Product4/2
  Add2/1 -> Product4/1
  Demux5/4 -> Gain21/1, Product6/3, Sign/1
  Sign/1 -> Product5/1
  Constant1/1 -> Add4/1
  Product5/1 -> Add4/2
  Add4/1 -> Abs/1, Sign1/1
  Sign1/1 -> Gain16/1
  Abs/1 -> Sqrt/1
  Gain16/1 -> Product6/1
  Sqrt/1 -> Product6/2
  Product4/1 -> Add5/2
  Add1/1 -> Gain1/1
  Gain1/1 -> Mux/2  "f14"
  Product6/1 -> Add5/1
  Add5/1 -> Mux/3  "f15"
  Gain21/1 -> Mux/4  "f16"
  Demux/2 -> Demux5/1
  In1/1 -> Demux/1
  Gain2/1 -> Mux/1
  Mux/1 -> Out1/1
  Demux/1 -> Demux9/1

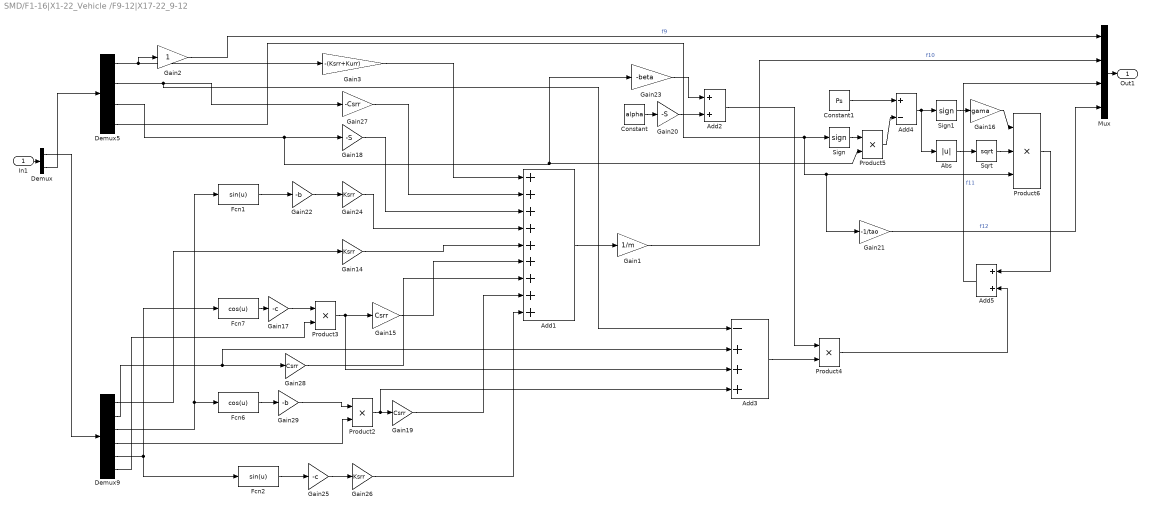
== system SMD/F1-16|X1-22_Vehicle /F9-12|X17-22_9-12 ==
  In1 : Inport
  Abs : Abs
  Add1 : Sum  Inputs=+++++++++
  Add2 : Sum
  Add3 : Sum  Inputs=-+++
  Add4 : Sum  Inputs=+-
  Add5 : Sum
  Constant : Constant  Value=alpha
  Constant1 : Constant  Value=Ps
  Demux : Demux  Outputs=2
  Demux5 : Demux
  Demux9 : Demux  Outputs=6
  Fcn1 : Fcn  Expr=sin(u)
  Fcn2 : Fcn  Expr=sin(u)
  Fcn6 : Fcn  Expr=cos(u)
  Fcn7 : Fcn  Expr=cos(u)
  Gain1 : Gain  Gain=1/m
  Gain14 : Gain  Gain=Ksrr
  Gain15 : Gain  Gain=Csrr
  Gain16 : Gain  Gain=gama
  Gain17 : Gain  Gain=-c
  Gain18 : Gain  Gain=-S
  Gain19 : Gain  Gain=Csrr
  Gain2 : Gain
  Gain20 : Gain  Gain=-S
  Gain21 : Gain  Gain=-1/tao
  Gain22 : Gain  Gain=-b
  Gain23 : Gain  Gain=-beta
  Gain24 : Gain  Gain=Ksrr
  Gain25 : Gain  Gain=-c
  Gain26 : Gain  Gain=Ksrr
  Gain27 : Gain  Gain=-Csrr
  Gain28 : Gain  Gain=Csrr
  Gain29 : Gain  Gain=-b
  Gain3 : Gain  Gain=-(Ksrr+Kurr)
  Mux : Mux
  Product{2..5} (4 alike) : Product
  Product6 : Product  Inputs=3
  Sign : Signum
  Sign1 : Signum
  Sqrt : Sqrt  SaturateOnIntegerOverflow=on
  Out1 : Outport
  wires:
  Demux5/1 -> Gain2/1, Gain3/1
  Demux9/1 -> Gain14/1
  Demux9/3 -> Fcn1/1, Fcn6/1
  Fcn1/1 -> Gain22/1
  Gain22/1 -> Gain24/1
  Demux9/5 -> Fcn2/1, Fcn7/1
  Fcn2/1 -> Gain25/1
  Gain25/1 -> Gain26/1
  Demux5/2 -> Add3/1, Gain27/1
  Demux9/2 -> Add3/2, Gain28/1
  Fcn6/1 -> Gain29/1
  Gain29/1 -> Product2/1
  Demux9/4 -> Product2/2
  Fcn7/1 -> Gain17/1
  Demux9/6 -> Product3/2
  Gain17/1 -> Product3/1
  Demux5/3 -> Gain23/1, Product5/2, Gain18/1
  Gain3/1 -> Add1/1
  Gain27/1 -> Add1/2
  Gain18/1 -> Add1/3
  Gain24/1 -> Add1/4
  Gain14/1 -> Add1/5
  Product3/1 -> Add3/3, Gain15/1
  Gain28/1 -> Add1/7
  Product2/1 -> Add3/4, Gain19/1
  Gain26/1 -> Add1/9
  Constant/1 -> Gain20/1
  Gain23/1 -> Add2/1
  Gain20/1 -> Add2/2
  Gain19/1 -> Add1/8
  Gain15/1 -> Add1/6
  Add3/1 -> Product4/2
  Add2/1 -> Product4/1
  Demux5/4 -> Gain21/1, Product6/3, Sign/1
  Sign/1 -> Product5/1
  Constant1/1 -> Add4/1
  Product5/1 -> Add4/2
  Add4/1 -> Abs/1, Sign1/1
  Sign1/1 -> Gain16/1
  Abs/1 -> Sqrt/1
  Gain16/1 -> Product6/1
  Sqrt/1 -> Product6/2
  Product4/1 -> Add5/2
  Add1/1 -> Gain1/1
  Gain2/1 -> Mux/1  "f9"
  Gain1/1 -> Mux/2  "f10"
  Product6/1 -> Add5/1
  Add5/1 -> Mux/3  "f11"
  Gain21/1 -> Mux/4  "f12"
  Mux/1 -> Out1/1
  Demux/1 -> Demux9/1
  In1/1 -> Demux/1
  Demux/2 -> Demux5/1

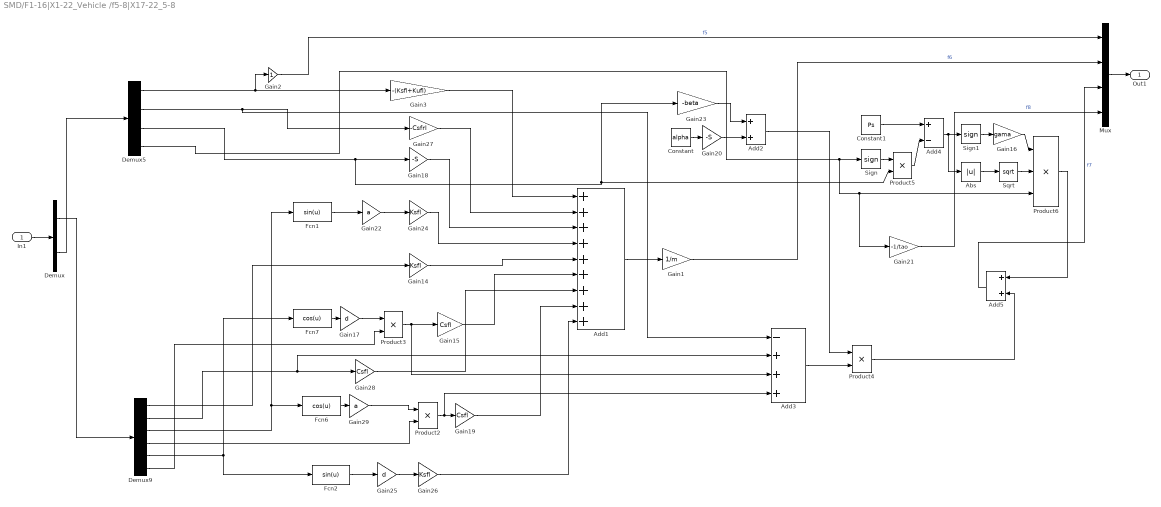
== system SMD/F1-16|X1-22_Vehicle /f5-8|X17-22_5-8 ==
  In1 : Inport
  Abs : Abs
  Add1 : Sum  Inputs=+++++++++
  Add2 : Sum
  Add3 : Sum  Inputs=-+++
  Add4 : Sum  Inputs=+-
  Add5 : Sum
  Constant : Constant  Value=alpha
  Constant1 : Constant  Value=Ps
  Demux : Demux  Outputs=2
  Demux5 : Demux
  Demux9 : Demux  Outputs=6
  Fcn1 : Fcn  Expr=sin(u)
  Fcn2 : Fcn  Expr=sin(u)
  Fcn6 : Fcn  Expr=cos(u)
  Fcn7 : Fcn  Expr=cos(u)
  Gain1 : Gain  Gain=1/m
  Gain14 : Gain  Gain=Ksfl
  Gain15 : Gain  Gain=Csfl
  Gain16 : Gain  Gain=gama
  Gain17 : Gain  Gain=d
  Gain18 : Gain  Gain=-S
  Gain19 : Gain  Gain=Csfl
  Gain2 : Gain
  Gain20 : Gain  Gain=-S
  Gain21 : Gain  Gain=-1/tao
  Gain22 : Gain  Gain=a
  Gain23 : Gain  Gain=-beta
  Gain24 : Gain  Gain=Ksfl
  Gain25 : Gain  Gain=d
  Gain26 : Gain  Gain=Ksfl
  Gain27 : Gain  Gain=-Csfrl
  Gain28 : Gain  Gain=Csfl
  Gain29 : Gain  Gain=a
  Gain3 : Gain  Gain=-(Ksfl+Kufl)
  Mux : Mux
  Product{2..5} (4 alike) : Product
  Product6 : Product  Inputs=3
  Sign : Signum
  Sign1 : Signum
  Sqrt : Sqrt  SaturateOnIntegerOverflow=on
  Out1 : Outport
  wires:
  Demux5/1 -> Gain2/1, Gain3/1
  Demux9/1 -> Gain14/1
  Demux9/3 -> Fcn1/1, Fcn6/1
  Fcn1/1 -> Gain22/1
  Gain22/1 -> Gain24/1
  Demux9/5 -> Fcn2/1, Fcn7/1
  Fcn2/1 -> Gain25/1
  Gain25/1 -> Gain26/1
  Demux5/2 -> Add3/1, Gain27/1
  Demux9/2 -> Add3/2, Gain28/1
  Fcn6/1 -> Gain29/1
  Gain29/1 -> Product2/1
  Demux9/4 -> Product2/2
  Fcn7/1 -> Gain17/1
  Demux9/6 -> Product3/2
  Gain17/1 -> Product3/1
  Demux5/3 -> Gain23/1, Product5/2, Gain18/1
  Gain3/1 -> Add1/1
  Gain27/1 -> Add1/2
  Gain18/1 -> Add1/3
  Gain24/1 -> Add1/4
  Gain14/1 -> Add1/5
  Product3/1 -> Add3/3, Gain15/1
  Gain28/1 -> Add1/7
  Product2/1 -> Add3/4, Gain19/1
  Gain26/1 -> Add1/9
  Constant/1 -> Gain20/1
  Gain23/1 -> Add2/1
  Gain20/1 -> Add2/2
  Gain19/1 -> Add1/8
  Gain15/1 -> Add1/6
  Add3/1 -> Product4/2
  Add2/1 -> Product4/1
  Demux5/4 -> Gain21/1, Product6/3, Sign/1
  Sign/1 -> Product5/1
  Constant1/1 -> Add4/1
  Product5/1 -> Add4/2
  Add4/1 -> Abs/1, Sign1/1
  Sign1/1 -> Gain16/1
  Abs/1 -> Sqrt/1
  Gain16/1 -> Product6/1
  Sqrt/1 -> Product6/2
  Product4/1 -> Add5/2
  Add1/1 -> Gain1/1
  Gain2/1 -> Mux/1  "f5"
  Gain1/1 -> Mux/2  "f6"
  Product6/1 -> Add5/1
  Add5/1 -> Mux/3  "f7"
  Gain21/1 -> Mux/4  "f8"
  Mux/1 -> Out1/1
  Demux/1 -> Demux9/1
  In1/1 -> Demux/1
  Demux/2 -> Demux5/1
